simulink model "Lab3_2_model"  (Simulink 7.4)
settings: Solver=ode4  SolverMode=SingleTasking  StartTime=0.0  StopTime=10.0  FixedStep=0.01  RelTol=1e-3
undefined symbols (not defined in the file or in its folder): A, Aplus, B, Bplus, C, Cplus, h
settings Model: Creator=adamus  LastModifiedBy=adamus
settings DataIOCC: LimitDataPoints=off

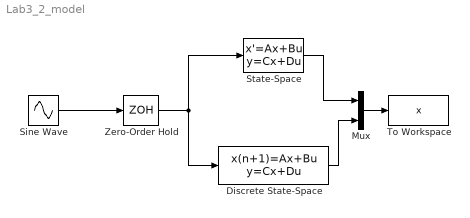
== system Lab3_2_model ==
  Discrete State-Space : DiscreteStateSpace  A=Aplus  B=Bplus  C=Cplus  D=0  X0=[1;1]  SampleTime=h
  Mux : Mux  Inputs=2
  Sine Wave : Sin  Amplitude=1  Bias=0  Frequency=1  Phase=0  Samples=10  SampleTime=0  Offset=0
  State-Space : StateSpace  A=A  B=B  C=C  D=0  X0=[1;1]
  To Workspace : ToWorkspace  VariableName=x  SampleTime=-1  SaveFormat=Array
  Zero-Order Hold : ZeroOrderHold  SampleTime=h
  wires:
  Sine Wave/1 -> Zero-Order Hold/1
  Zero-Order Hold/1 -> State-Space/1, Discrete State-Space/1
  Mux/1 -> To Workspace/1
  State-Space/1 -> Mux/1
  Discrete State-Space/1 -> Mux/2
